simulink model "ClosedBoxLS_MDL"  (R2021a)
settings: Solver=VariableStepAuto  StartTime=0.0  StopTime=tmax  RelTol=1e-3
undefined symbols (not defined in the file or in its folder): a0, a1, a2, b0, b1, b2, Bl, Cmc, Mms, Rms, Sd, tau, ts
libraries: simulink x1
settings Model: Creator=padlewsk  LastModifiedBy=padlewsk
settings DataIOCC: ReturnWorkspaceOutputs=off

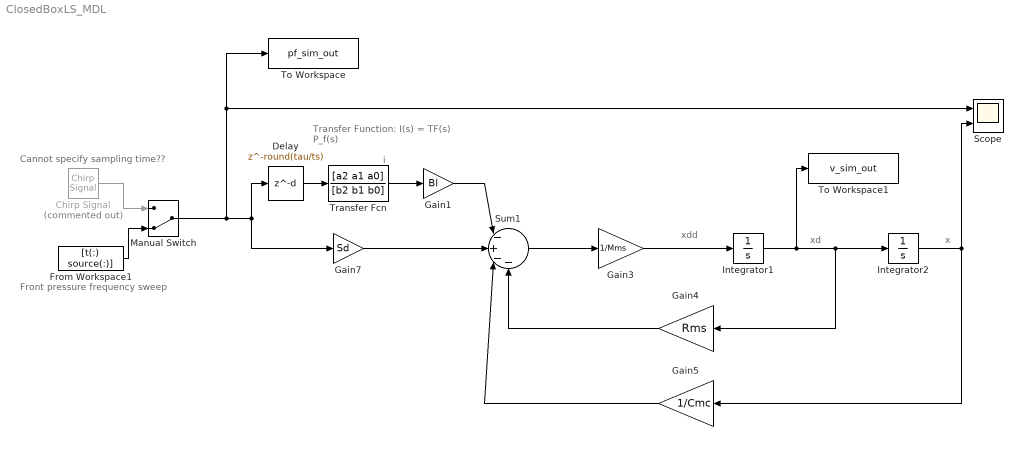
== system ClosedBoxLS_MDL ==
  note: Front pressure frequency sweep
  note: xd
  note: xdd
  note: x
  note: i
  note: Transfer Function:
      |   I(s) = TF(s) P_f(s)
  note: Cannot specify sampling time??
  Chirp Signal : simulink/Sources/Chirp Signal  Commented=on  f1=fi  T=tf  f2=ff
  Delay : Delay  DelayLength=round(tau/ts)
  From Workspace1 : FromWorkspace  VariableName=[t(:) source(:)]  SampleTime=ts
  Gain1 : Gain  Gain=Bl
  Gain3 : Gain  Gain=1/Mms
  Gain4 : Gain  Gain=Rms
  Gain5 : Gain  Gain=1/Cmc
  Gain7 : Gain  Gain=Sd
  Integrator1 : Integrator
  Integrator2 : Integrator
  Manual Switch : ManualSwitch  CurrentSetting=0
  Scope : Scope  NumInputPorts=2
  Sum1 : Sum  Inputs=|-+--
  To Workspace : ToWorkspace  VariableName=pf_sim_out  SaveFormat=Timeseries  SampleTime=-1
  To Workspace1 : ToWorkspace  VariableName=v_sim_out  SaveFormat=Timeseries  SampleTime=-1
  Transfer Fcn : TransferFcn  Numerator=[a2 a1 a0]  Denominator=[b2 b1 b0]
  wires:
  Gain1/1 -> Sum1/1
  Integrator2/1 -> Scope/2, Gain5/1
  Sum1/1 -> Gain3/1
  Gain3/1 -> Integrator1/1
  Gain4/1 -> Sum1/4
  Gain5/1 -> Sum1/3
  Gain7/1 -> Sum1/2
  Transfer Fcn/1 -> Gain1/1
  Chirp Signal/1 -> Manual Switch/1
  From Workspace1/1 -> Manual Switch/2
  Manual Switch/1 -> To Workspace/1, Scope/1, Delay/1, Gain7/1
  Integrator1/1 -> To Workspace1/1, Integrator2/1, Gain4/1
  Delay/1 -> Transfer Fcn/1
